simulink model "Balancer_pos_p2p"  (R2025b)
settings: Solver=VariableStepAuto  StartTime=0.0  StopTime=12  FixedStep=0.01  RelTol=1e-3
undefined symbols (not defined in the file or in its folder): X, Y, Z
libraries: sm_lib x26, nesl_utility x13, slpidlib x1
(part 2 of 2)

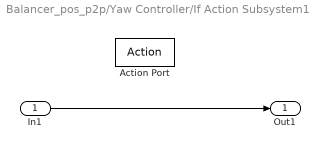
== system Balancer_pos_p2p/Yaw Controller/If Action Subsystem1 ==
  In1 : Inport
  Action Port : ActionPort  ActionPortLabel=if(u1 > 0)
  Out1 : Outport
  wires:
  In1/1 -> Out1/1

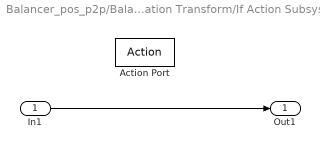
== system Balancer_pos_p2p/Balancer/Rotation Transform/If Action Subsystem ==
  In1 : Inport
  Action Port : ActionPort  ActionPortLabel=if(u1 > 0)
  Out1 : Outport
  wires:
  In1/1 -> Out1/1

== system Balancer_pos_p2p/Balancer/Rotation Transform/If Action Subsystem1 ==
  In1 : Inport
  Action Port : ActionPort  ActionPortLabel=else
  Out1 : Outport
  wires:
  In1/1 -> Out1/1

== system Balancer_pos_p2p/Balancer/Rotation Transform/If Action Subsystem2 ==
  Y rotation : Inport
  Action Port : ActionPort  ActionPortLabel=if(u1 > 0)
  Out1 : Outport
  wires:
  Y rotation/1 -> Out1/1

== system Balancer_pos_p2p/Balancer/Rotation Transform/If Action Subsystem3 ==
  X rotation : Inport
  Action Port : ActionPort  ActionPortLabel=else
  Out1 : Outport
  wires:
  X rotation/1 -> Out1/1

== matlab function Balancer_pos_p2p/MATLAB Function ==
  data: p_end output; v_max output; a_max output
function [p_end,v_max,a_max] = fcn
%#codegen
p_end=0.15;%
v_max=0.08;%
a_max=0.08;%
